simulink model "Differential_robot_dynamic_model"  (R2024b)
settings: Solver=VariableStepAuto  StartTime=0.0  StopTime=10.0  RelTol=1e-3
values from neighbouring files (symbols this model uses):
  J = 0.1    [Init_parameters_Dynamic.m]
  L = 150e-3    (= 0.15)    [Init_parameters_Dynamic.m]    (also in Init_parameters_kinematic.m)
  m = 1.0    (= 1)    [Init_parameters_Dynamic.m]
  omega = 0    [Init_parameters_Dynamic.m]
  r = 25e-3    (= 0.025)    [Init_parameters_Dynamic.m]    (also in Init_parameters_kinematic.m)
  theta = 0    [Init_parameters_Dynamic.m]    (also in Init_parameters_kinematic.m)
  v = 0    [Init_parameters_Dynamic.m]
  x = 0    [Init_parameters_Dynamic.m]    (also in Init_parameters_kinematic.m)
  y = 0    [Init_parameters_Dynamic.m]    (also in Init_parameters_kinematic.m)
libraries: simulink_extras x1
settings Model: Creator=Nabil  LastModifiedBy=Nabil

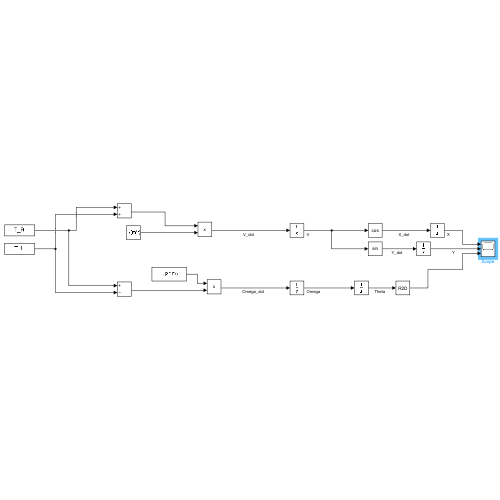
[thumbnail: Simulink's stored preview of the top-level diagram]
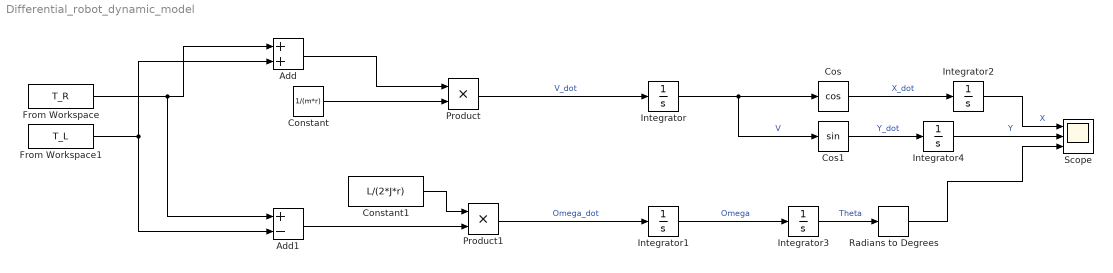
== system Differential_robot_dynamic_model ==
  Add : Sum
  Add1 : Sum  Inputs=+-
  Constant : Constant  Value=1/(m*r)
  Constant1 : Constant  Value=L/(2*J*r)
  Cos : Trigonometry  Operator=cos
  Cos1 : Trigonometry
  From Workspace : FromWorkspace  VariableName=T_R
  From Workspace1 : FromWorkspace  VariableName=T_L
  Integrator : Integrator  InitialCondition=v
  Integrator1 : Integrator  InitialCondition=omega
  Integrator2 : Integrator  InitialCondition=x
  Integrator3 : Integrator  InitialCondition=theta
  Integrator4 : Integrator  InitialCondition=y
  Product : Product
  Product1 : Product
  Radians to Degrees : simulink_extras/Transformations/Radians to Degrees
  Scope : Scope  NumInputPorts=3
  wires:
  Product/1 -> Integrator/1  "V_dot"
  Add/1 -> Product/1
  Constant/1 -> Product/2
  Constant1/1 -> Product1/1
  Integrator/1 -> Cos1/1, Cos/1  "V"
  Integrator1/1 -> Integrator3/1  "Omega"
  Product1/1 -> Integrator1/1  "Omega_dot"
  Add1/1 -> Product1/2
  From Workspace/1 -> Add1/1, Add/1
  From Workspace1/1 -> Add1/2, Add/2
  Cos/1 -> Integrator2/1  "X_dot"
  Cos1/1 -> Integrator4/1  "Y_dot"
  Integrator3/1 -> Radians to Degrees/1  "Theta"
  Integrator4/1 -> Scope/2  "Y"
  Integrator2/1 -> Scope/1  "X"
  Radians to Degrees/1 -> Scope/3
